simulink model "LinearizationPartb"  (R2020a)
settings: Solver=VariableStepAuto  StartTime=0.0  StopTime=sim_time  RelTol=1e-3
values from neighbouring files (symbols this model uses):
  C_0 = 0.5    [Linearization.m]
  gamma = 0.1    [Linearization.m]
  Lc = 5    [Linearization.m]
  N = 20    [Linearization.m]
  sigma = 5    [Linearization.m]
  v_0 = 0.1    [Linearization.m]
settings Model: Creator=sangmin  LastModifiedBy=sangmin
settings DataIOCC: ReturnWorkspaceOutputs=off

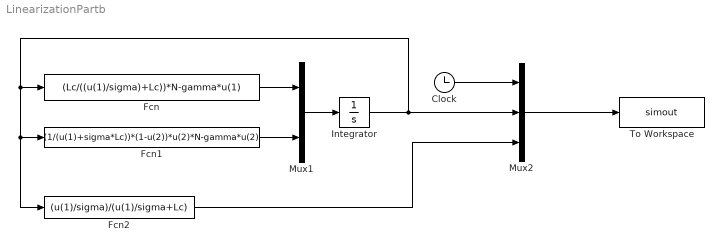
== system LinearizationPartb ==
  Clock : Clock
  Fcn : Fcn  Expr=(Lc/((u(1)/sigma)+Lc))*N-gamma*u(1)
  Fcn1 : Fcn  Expr=(1/(u(1)+sigma*Lc))*(1-u(2))*u(2)*N-gamma*u(2)
  Fcn2 : Fcn  Expr=(u(1)/sigma)/(u(1)/sigma+Lc)
  Integrator : Integrator  InitialCondition=[C_0 ; v_0]
  Mux1 : Mux  Inputs=2
  Mux2 : Mux  Inputs=3
  To Workspace : ToWorkspace  VariableName=simout  SampleTime=-1
  wires:
  Integrator/1 -> Fcn2/1, Fcn1/1, Fcn/1, Mux2/2
  Fcn/1 -> Mux1/1
  Fcn1/1 -> Mux1/2
  Mux1/1 -> Integrator/1
  Clock/1 -> Mux2/1
  Mux2/1 -> To Workspace/1
  Fcn2/1 -> Mux2/3
